simulink subsystem "LED_sub"  (R2023b)
settings: Solver=VariableStepAuto  StartTime=0.0  StopTime=10.0  RelTol=1e-3
libraries: arduinolib x3, simulink x1
settings Model: Creator=alumnos  LastModifiedBy=Usuario_UMA

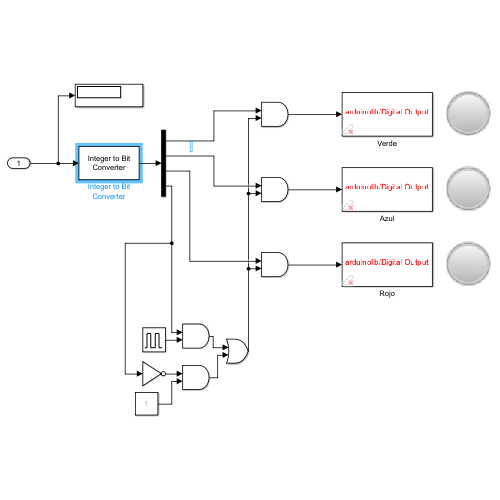
[thumbnail: Simulink's stored preview of the top-level diagram]
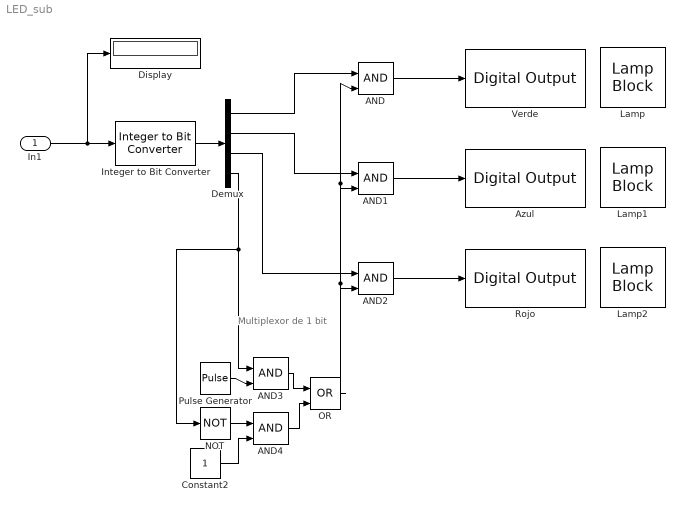
== system LED_sub ==
  note: Multiplexor de 1 bit
  In1 : Inport
  AND{,1..4} (5 alike) : Logic  IconShape=distinctive  AllPortsSameDT=off  OutDataTypeStr=boolean
  Azul : arduinolib/Digital Output  pinNumber=53  Direction=output  blockPlatform=arduino
  Constant2 : Constant
  Demux : Demux
  Display : Display
  Integer to Bit Converter : simulink/Logic and Bit Operations/Integer to Bit Converter  nbits=4  signedInputValues=Unsigned  bitOrder=MSB first  outDtype=boolean
  Lamp : LampBlock  LabelPosition=Hide
  Lamp1 : LampBlock  LabelPosition=Hide
  Lamp2 : LampBlock  LabelPosition=Hide
  NOT : Logic  Operator=NOT  IconShape=distinctive  AllPortsSameDT=off  OutDataTypeStr=boolean
  OR : Logic  Operator=OR  IconShape=distinctive  AllPortsSameDT=off  OutDataTypeStr=boolean
  Pulse Generator : DiscretePulseGenerator  PulseType=Time based  Period=1  PulseWidth=50
  Rojo : arduinolib/Digital Output  pinNumber=49  Direction=output  blockPlatform=arduino
  Verde : arduinolib/Digital Output  pinNumber=51  Direction=output  blockPlatform=arduino
  wires:
  AND3/1 -> OR/1
  NOT/1 -> AND4/1
  Constant2/1 -> AND4/2
  OR/1 -> AND/2, AND1/2, AND2/2
  In1/1 -> Display/1, Integer to Bit Converter/1
  Demux/1 -> AND/1
  Integer to Bit Converter/1 -> Demux/1
  AND/1 -> Verde/1
  Pulse Generator/1 -> AND3/2
  Demux/4 -> NOT/1, AND3/1
  AND4/1 -> OR/2
  AND1/1 -> Azul/1
  AND2/1 -> Rojo/1
  Demux/2 -> AND1/1
  Demux/3 -> AND2/1
